simulink model "Test_harness"  (R2025b)
settings: Solver=FixedStepDiscrete  StartTime=0.0  StopTime=25  FixedStep=0.01  RelTol=1e-3
undefined symbols (not defined in the file or in its folder): delta, wc
settings Model: Creator=lenovo  LastModifiedBy=lenovo

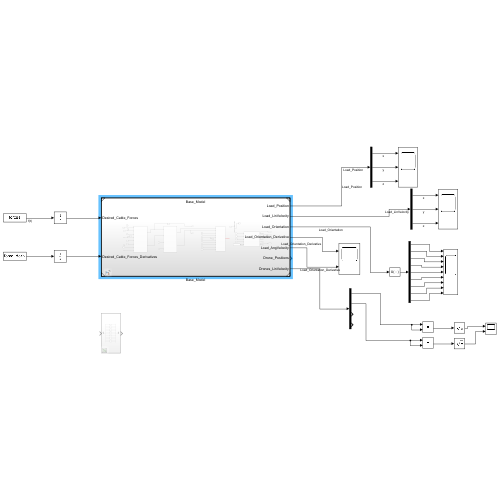
[thumbnail: Simulink's stored preview of the top-level diagram]
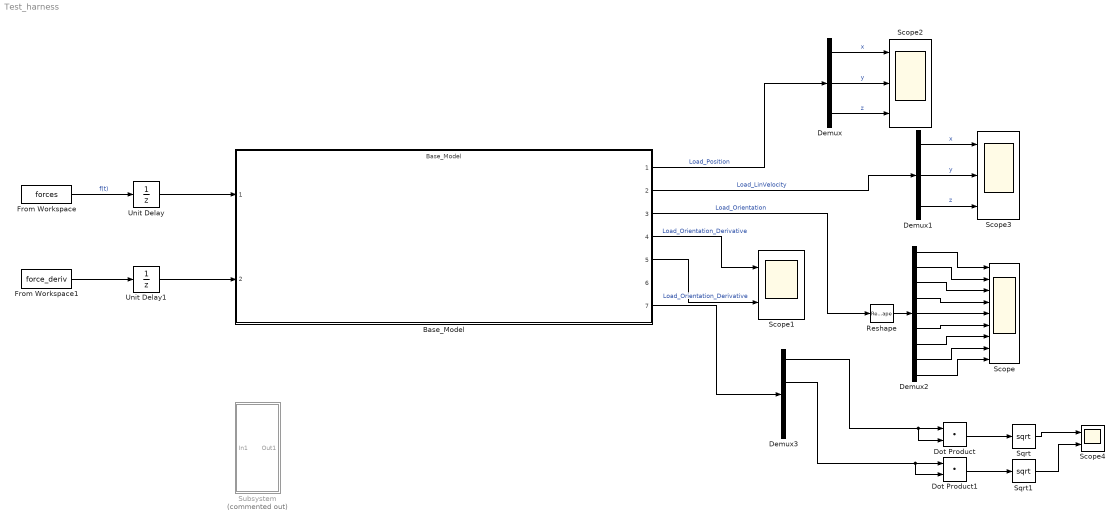
== system Test_harness ==
  Base_Model : ModelReference  ModelNameDialog=Base_Model.slx  SimulationMode=Normal  ModelReferenceVersion=1.70
  Demux : Demux  Outputs=3
  Demux1 : Demux  Outputs=3
  Demux2 : Demux  Outputs=9
  Demux3 : Demux
  Dot Product : DotProduct  OutDataTypeStr=Inherit: Inherit via internal rule
  Dot Product1 : DotProduct  OutDataTypeStr=Inherit: Inherit via internal rule
  From Workspace : FromWorkspace  VariableName=forces  OutputAfterFinalValue=Holding final value
  From Workspace1 : FromWorkspace  VariableName=force_deriv  OutputAfterFinalValue=Holding final value
  Reshape : Reshape
  Scope : Scope  NumInputPorts=9
      settings: ActiveDisplayYMinimum=0.9  ActiveDisplayYMaximum=1.1
  Scope1 : Scope  NumInputPorts=2
  Scope2 : Scope  NumInputPorts=3
      settings: ActiveDisplayYMinimum=-0.895178181091243  ActiveDisplayYMaximum=8.05660362982119  DataLoggingVariableName=Load_x1
  Scope3 : Scope  NumInputPorts=3
      settings: ActiveDisplayYMinimum=-1  ActiveDisplayYMaximum=1  DataLoggingVariableName=Load_x2
  Scope4 : Scope  NumInputPorts=2
      settings: ActiveDisplayYMinimum=-1.9423704031655016  ActiveDisplayYMaximum=17.481333628489519  DataLoggingVariableName=ScopeData2
  Sqrt : Sqrt
  Sqrt1 : Sqrt
  Subsystem : Subsystem  Commented=on
  Unit Delay : UnitDelay  SampleTime=-1  HasFrameUpgradeWarning=on
  Unit Delay1 : UnitDelay  SampleTime=-1  HasFrameUpgradeWarning=on
  wires:
  Base_Model/1 -> Demux/1  "Load_Position"
  Base_Model/3 -> Reshape/1  "Load_Orientation"
  Base_Model/4 -> Scope1/1  "Load_Orientation_Derivative"
  Base_Model/5 -> Scope1/2  "Load_Orientation_Derivative"
  Demux/1 -> Scope2/1  "x"
  Demux/2 -> Scope2/2  "y"
  Demux/3 -> Scope2/3  "z"
  From Workspace1/1 -> Unit Delay1/1
  Demux1/3 -> Scope3/3  "z"
  Demux1/2 -> Scope3/2  "y"
  Demux1/1 -> Scope3/1  "x"
  Base_Model/2 -> Demux1/1  "Load_LinVelocity"
  Unit Delay1/1 -> Base_Model/2
  From Workspace/1 -> Unit Delay/1  "f(t)"
  Unit Delay/1 -> Base_Model/1
  Demux2/1 -> Scope/1
  Demux2/2 -> Scope/2
  Demux2/3 -> Scope/3
  Demux2/4 -> Scope/4
  Demux2/5 -> Scope/5
  Demux2/6 -> Scope/6
  Demux2/7 -> Scope/7
  Demux2/8 -> Scope/8
  Demux2/9 -> Scope/9
  Reshape/1 -> Demux2/1
  Base_Model/7 -> Demux3/1
  Demux3/1 -> Dot Product/1, Dot Product/2
  Dot Product/1 -> Sqrt/1
  Sqrt/1 -> Scope4/1
  Sqrt1/1 -> Scope4/2
  Dot Product1/1 -> Sqrt1/1
  Demux3/2 -> Dot Product1/2, Dot Product1/1

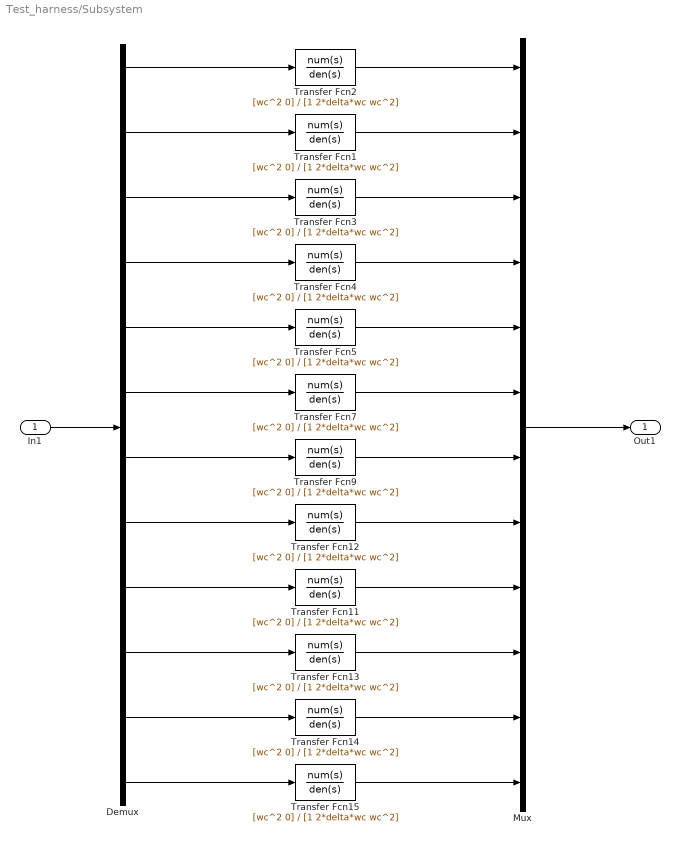
== system Test_harness/Subsystem ==
  In1 : Inport
  Demux : Demux  Outputs=12
  Mux : Mux  Inputs=12
  Transfer Fcn{1..5,7,9,11..15} (12 alike) : TransferFcn  Numerator=[wc^2 0]  Denominator=[1 2*delta*wc wc^2]
  Out1 : Outport
  wires:
  Demux/1 -> Transfer Fcn2/1
  Demux/2 -> Transfer Fcn1/1
  Demux/3 -> Transfer Fcn3/1
  Demux/4 -> Transfer Fcn4/1
  Demux/5 -> Transfer Fcn5/1
  Demux/6 -> Transfer Fcn7/1
  Demux/7 -> Transfer Fcn9/1
  Demux/8 -> Transfer Fcn12/1
  Demux/9 -> Transfer Fcn11/1
  Demux/10 -> Transfer Fcn13/1
  Demux/11 -> Transfer Fcn14/1
  Demux/12 -> Transfer Fcn15/1
  Transfer Fcn2/1 -> Mux/1
  Transfer Fcn1/1 -> Mux/2
  Transfer Fcn3/1 -> Mux/3
  Transfer Fcn4/1 -> Mux/4
  Transfer Fcn5/1 -> Mux/5
  Transfer Fcn7/1 -> Mux/6
  Transfer Fcn9/1 -> Mux/7
  Transfer Fcn12/1 -> Mux/8
  Transfer Fcn11/1 -> Mux/9
  Transfer Fcn13/1 -> Mux/10
  Transfer Fcn14/1 -> Mux/11
  Transfer Fcn15/1 -> Mux/12
  In1/1 -> Demux/1
  Mux/1 -> Out1/1
